simulink model "Swarm_Offline"  (Simulink 7.7)
settings: Solver=ode5  StartTime=0.0  StopTime=inf  FixedStep=sample_time  RelTol=1e-3
InitFcn:
  | sample_time=0.005;%0.004;%0.0025;%0.02;
  | sample_time_Vicon = 0.005;
  | DeltaT = 0.02;
  | g = 9.81;
  | H0 = g%0.3165;
  | Kl = 1;
  | 
  | Q6_mass = 0.73;
  | 
  | Q6_Omega_r = 1.5; %for horizon ref
  | Q6_Zeta_r = 0.5; %for horizon ref
  | Q6_Omega_r_h = 2;%for vertical ref
  | Q6_Zeta_r_h = 1; %for vertical ref
  | 
  | Q6_Omega = 1.5; %for horizon control
  | Q6_Zeta = 0.5; %for horizon control
  | Q6_Omega_h= 2; %for vertical control
  | Q6_Zeta_h = 0.7; %for vertical control
  | 
  | Q6_acc_max = 5;%horizontal max acc
  | Q6_acc_max_h = 3;%horizontal max acc
  | 
  | omega_circle = 36*pi/180;
  | omega_h = 0.1;%Ascending speed
  | PI = pi;
  | Circle_R = 2;
  | MAX_Height = -1;
  | 
  | r0=2; %desired separation distance
  | num = 3; %number of neighbors
  | 
  | load UAV1.mat
  | load UAV2.mat
  | load UAV3.mat
  | load UAV4.mat
libraries: X330_Control x22, simulink x16
(part 3 of 3)

== matlab function Agent 4/Swarming/swarm/2 UAV Swarm Algorithm ==
  data: w output double; pos1 input double; pos_cmd1 output double; pos2 input double; r0 input double
function [w,pos_cmd1] = fcn(pos1,pos2,r0)

% Swarm algorithm for Vicon environment. 
% Heading concensus is not considered, only positions. 
% Hence, only the inter-agent potential in terms of separation distance is
% taken into consideration. 
%
% Adapted from func_swarm_2UAV_2D_decentralized.m

% 25 Apr 2011

%r0 = 2;   % desired separation

delta = pos2(1:2) - pos1(1:2);
b   = 0.1;
pos_cmd1 = zeros(4,1);
w = 0;

r = norm(delta) - r0;                 % relative distance

if abs(r) < b
    w = 0;
else if r > b
    w = (2/(1+exp(-4*(r-b)))-1)*1;          % potential, max value at r=1.5m
    else if r < -b
            w = (2/(1+exp(-4*(r+b)))-1)*1;
        end
    end
end                                       % scaled by 1.0

theta = atan2(delta(2),delta(1));

pos_cmd1(1) = w*cos(theta);
pos_cmd1(2) = w*sin(theta);

% vel_cmd2(1) = -w*cos(theta);  
% vel_cmd2(2) = -w*sin(theta);

== matlab function Agent 4/Swarming/swarm1/2 UAV Swarm Algorithm ==
  data: w output double; pos1 input double; pos_cmd1 output double; pos2 input double; r0 input double
function [w,pos_cmd1] = fcn(pos1,pos2,r0)

% Swarm algorithm for Vicon environment. 
% Heading concensus is not considered, only positions. 
% Hence, only the inter-agent potential in terms of separation distance is
% taken into consideration. 
%
% Adapted from func_swarm_2UAV_2D_decentralized.m

% 25 Apr 2011

%r0 = 2;   % desired separation

delta = pos2(1:2) - pos1(1:2);
b   = 0.1;
pos_cmd1 = zeros(4,1);
w = 0;

r = norm(delta) - r0;                 % relative distance

if abs(r) < b
    w = 0;
else if r > b
    w = (2/(1+exp(-4*(r-b)))-1)*1;          % potential, max value at r=1.5m
    else if r < -b
            w = (2/(1+exp(-4*(r+b)))-1)*1;
        end
    end
end                                       % scaled by 1.0

theta = atan2(delta(2),delta(1));

pos_cmd1(1) = w*cos(theta);
pos_cmd1(2) = w*sin(theta);

% vel_cmd2(1) = -w*cos(theta);  
% vel_cmd2(2) = -w*sin(theta);

== matlab function Agent 4/Swarming/swarm2/2 UAV Swarm Algorithm ==
  data: w output double; pos1 input double; pos_cmd1 output double; pos2 input double; r0 input double
function [w,pos_cmd1] = fcn(pos1,pos2,r0)

% Swarm algorithm for Vicon environment. 
% Heading concensus is not considered, only positions. 
% Hence, only the inter-agent potential in terms of separation distance is
% taken into consideration. 
%
% Adapted from func_swarm_2UAV_2D_decentralized.m

% 25 Apr 2011

%r0 = 2;   % desired separation

delta = pos2(1:2) - pos1(1:2);
b   = 0.1;
pos_cmd1 = zeros(4,1);
w = 0;

r = norm(delta) - r0;                 % relative distance

if abs(r) < b
    w = 0;
else if r > b
    w = (2/(1+exp(-4*(r-b)))-1)*1;          % potential, max value at r=1.5m
    else if r < -b
            w = (2/(1+exp(-4*(r+b)))-1)*1;
        end
    end
end                                       % scaled by 1.0

theta = atan2(delta(2),delta(1));

pos_cmd1(1) = w*cos(theta);
pos_cmd1(2) = w*sin(theta);

% vel_cmd2(1) = -w*cos(theta);  
% vel_cmd2(2) = -w*sin(theta);
